simulink model "Simulation"  (Simulink 7.4)
settings: Solver=ode45  StartTime=0.0  StopTime=30.0  MaxStep=0.2  RelTol=1e-3
PostLoadFcn:
  | load StoryboardBus.mat
libraries: RailCab x2
settings Model: Creator=dread  LastModifiedBy=dread

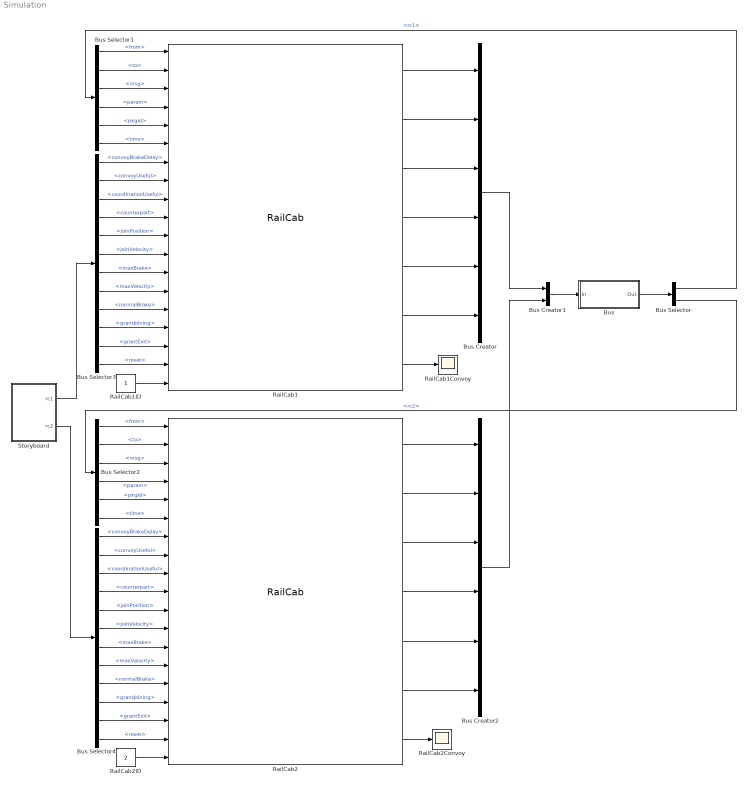
== system Simulation ==
  Bus : Subsystem
  Bus Creator : BusCreator  Inputs=6  UseBusObject=on
      settings: BusObject=PacketBus
  Bus Creator1 : BusCreator  Inputs=2  UseBusObject=on
      settings: BusObject=RailCabBus
  Bus Creator2 : BusCreator  Inputs=6  UseBusObject=on
      settings: BusObject=PacketBus
  Bus Selector : BusSelector  OutputSignals=rc1,rc2
  Bus Selector1 : BusSelector  OutputSignals=from,to,msg,param,pkgid,time
  Bus Selector2 : BusSelector  OutputSignals=from,to,msg,param,pkgid,time
  Bus Selector3 : BusSelector  OutputSignals=convoyBrakeDelay,convoyUseful,coordinationUseful,counterpart,joinPosition,joinVelocity,maxBrake,maxVelocity,normalBrake,grantJoining,grantExit,reset
  Bus Selector4 : BusSelector  OutputSignals=convoyBrakeDelay,convoyUseful,coordinationUseful,counterpart,joinPosition,joinVelocity,maxBrake,maxVelocity,normalBrake,grantJoining,grantExit,reset
  RailCab1 : RailCab/RailCab  SystemSampleTime=-1
  RailCab1Convoy : Scope
      settings: TimeRange=30
  RailCab1ID : Constant  OutDataTypeMode=uint8  OutDataType=fixdt(1, 16)  OutScaling=2^0  OutDataTypeStr=uint8
  RailCab2 : RailCab/RailCab  SystemSampleTime=-1
  RailCab2Convoy : Scope
  RailCab2ID : Constant  Value=2  OutDataTypeMode=uint8  OutDataType=fixdt(1, 16)  OutScaling=2^0  OutDataTypeStr=uint8
  Storyboard : Subsystem
  wires:
  Bus/1(Out) -> Bus Selector/1
  Bus Selector/1 -> Bus Selector1/1  "<rc1>"
  Bus Creator/1 -> Bus Creator1/1
  Bus Creator1/1 -> Bus/1(In)
  Bus Creator2/1 -> Bus Creator1/2
  Bus Selector/2 -> Bus Selector2/1  "<rc2>"
  Storyboard/1(rc1) -> Bus Selector3/1
  Storyboard/2(rc2) -> Bus Selector4/1
  Bus Selector3/1 -> RailCab1/7  "<convoyBrakeDelay>"
  Bus Selector3/2 -> RailCab1/8  "<convoyUseful>"
  Bus Selector3/3 -> RailCab1/9  "<coordinationUseful>"
  Bus Selector3/4 -> RailCab1/10  "<counterpart>"
  Bus Selector3/5 -> RailCab1/11  "<joinPosition>"
  Bus Selector3/6 -> RailCab1/12  "<joinVelocity>"
  Bus Selector3/7 -> RailCab1/13  "<maxBrake>"
  Bus Selector3/8 -> RailCab1/14  "<maxVelocity>"
  Bus Selector3/9 -> RailCab1/15  "<normalBrake>"
  Bus Selector3/10 -> RailCab1/16  "<grantJoining>"
  Bus Selector3/11 -> RailCab1/17  "<grantExit>"
  Bus Selector3/12 -> RailCab1/18  "<reset>"
  Bus Selector1/1 -> RailCab1/1  "<from>"
  Bus Selector1/2 -> RailCab1/2  "<to>"
  Bus Selector1/3 -> RailCab1/3  "<msg>"
  Bus Selector1/4 -> RailCab1/4  "<param>"
  Bus Selector1/5 -> RailCab1/5  "<pkgid>"
  Bus Selector1/6 -> RailCab1/6  "<time>"
  RailCab1/1 -> Bus Creator/1
  RailCab1/2 -> Bus Creator/2
  RailCab1/3 -> Bus Creator/3
  RailCab1/4 -> Bus Creator/4
  RailCab1/5 -> Bus Creator/5
  RailCab1/6 -> Bus Creator/6
  RailCab1ID/1 -> RailCab1/19
  Bus Selector2/1 -> RailCab2/1  "<from>"
  Bus Selector2/2 -> RailCab2/2  "<to>"
  Bus Selector2/3 -> RailCab2/3  "<msg>"
  Bus Selector2/4 -> RailCab2/4  "<param>"
  Bus Selector2/5 -> RailCab2/5  "<pkgid>"
  Bus Selector2/6 -> RailCab2/6  "<time>"
  Bus Selector4/1 -> RailCab2/7  "<convoyBrakeDelay>"
  Bus Selector4/2 -> RailCab2/8  "<convoyUseful>"
  Bus Selector4/3 -> RailCab2/9  "<coordinationUseful>"
  Bus Selector4/4 -> RailCab2/10  "<counterpart>"
  Bus Selector4/5 -> RailCab2/11  "<joinPosition>"
  Bus Selector4/6 -> RailCab2/12  "<joinVelocity>"
  Bus Selector4/7 -> RailCab2/13  "<maxBrake>"
  Bus Selector4/8 -> RailCab2/14  "<maxVelocity>"
  Bus Selector4/9 -> RailCab2/15  "<normalBrake>"
  Bus Selector4/10 -> RailCab2/16  "<grantJoining>"
  Bus Selector4/11 -> RailCab2/17  "<grantExit>"
  Bus Selector4/12 -> RailCab2/18  "<reset>"
  RailCab2ID/1 -> RailCab2/19
  RailCab2/1 -> Bus Creator2/1
  RailCab2/2 -> Bus Creator2/2
  RailCab2/3 -> Bus Creator2/3
  RailCab2/4 -> Bus Creator2/4
  RailCab2/5 -> Bus Creator2/5
  RailCab2/6 -> Bus Creator2/6
  RailCab1/7 -> RailCab1Convoy/1
  RailCab2/7 -> RailCab2Convoy/1

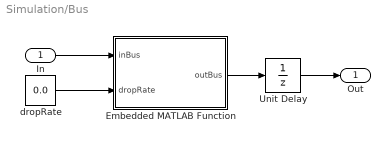
== system Simulation/Bus ==
  In : Inport  OutDataType=CommunicationBus
  Embedded MATLAB Function : Stateflow chart
  Unit Delay : UnitDelay  SampleTime=-1
  dropRate : Constant  Value=0.0  OutDataTypeMode=double  OutDataType=fixdt(1, 16)  OutScaling=2^0  OutDataTypeStr=double
  Out : Outport  OutDataType=CommunicationBus
  wires:
  Unit Delay/1 -> Out/1
  Embedded MATLAB Function/1(outBus) -> Unit Delay/1
  In/1 -> Embedded MATLAB Function/1(inBus)
  dropRate/1 -> Embedded MATLAB Function/2(dropRate)

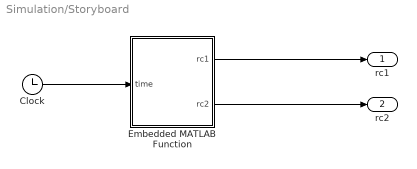
== system Simulation/Storyboard ==
  Clock : Clock
      settings: Decimation=10
  Embedded MATLAB Function : Stateflow chart
  rc1 : Outport  OutDataType=fixdt(1, 16)  OutScaling=2^0
  rc2 : Outport  Port=2  OutDataType=fixdt(1, 16)  OutScaling=2^0
  wires:
  Embedded MATLAB Function/1(rc1) -> rc1/1
  Embedded MATLAB Function/2(rc2) -> rc2/1
  Clock/1 -> Embedded MATLAB Function/1(time)

== matlab function Bus/Embedded MATLAB Function ==
  data: inBus input Bus: RailCabBus; outBus output Bus: RailCabBus; dropRate input double [0..1]
function outBus = BusImpl(inBus, dropRate)
%#eml
eml.extrinsic('fieldnames','disp','setfield','fprintf');

queueSize = 10; %length of queue
numShuttles = 0; %Define data type
numShuttles = numel(fieldnames(inBus)); %Shuttles connected to the bus
assert(numShuttles <= 20) %Defines an upper bound for number of shuttles. 
%Important for static memory allocation. 

%We need persistent queues
persistent queue

%Initialize the queues
if isempty(queue)
    queue = repmat(emptyPacket(), numShuttles, queueSize);
end

%Clean outbus
outBus = inBus;
for i = 1:numShuttles
    outBus = setfield(outBus, createRailCabName(i), emptyPacket());
end

%Retrieve packets
for i = 1:numShuttles
    packet = getPacketFromRC(inBus, i);
    if isValid(packet, numShuttles) 
        if ~dropPacket(dropRate)
            target = packet.to;
            queue(target,:) = enqueue(queue(target,:), packet);
        end
    end
end

%Send packet from queue
for i = 1:numShuttles
    if ~isEmpty(queue(i,:))
        
        %Debug: Print messages except ACK        
%         packet = front(queue(i,:));
%         if packet.msg ~= 255 %No ACK
%             fprintf('%3u: %u->%u :%3u (%.1f) @%.2f\n', packet.pkgid, packet.from, packet.to, packet.msg, packet.param, packet.time);
%         end
        
        outBus = sendPacket(outBus, front(queue(i,:)));
        queue(i,:) = dequeue(queue(i,:));                
    end    
end

%%%%%%%%%%%%%%%%%%%%%%%%%%%%%%%%%%%%%%%%%%%%%%%%%%%%%%%%%%%%%%%%%%%%%%%%%%%
%% BUS
%%%%%%%%%%%%%%%%%%%%%%%%%%%%%%%%%%%%%%%%%%%%%%%%%%%%%%%%%%%%%%%%%%%%%%%%%%%

function name = createRailCabName(index) %#eml
%Create name for the railcab used on the bus
eml.extrinsic('sprintf');
name = sprintf('rc%d', index);

function packet = getPacketFromRC(inBus, index) %#eml
%Retrieve a packet from a railcab
eml.extrinsic('getfield');
packet = emptyPacket();
packet = getfield(inBus,createRailCabName(index));

function outBus = sendPacket(outBusIn, packet) %#eml
%Send a packet to a railcab
eml.extrinsic('setfield','getfield');
outBusIn = setfield(outBusIn,createRailCabName(packet.to),packet);
outBus = outBusIn;

function drop = dropPacket(dropRate) %#eml
%Compute whether to drop the packet or not according to the given rate
eml.extrinsic('exprnd');
rand = 0;
rand = exprnd(1);
drop = rand  < -log(1-dropRate);


%%%%%%%%%%%%%%%%%%%%%%%%%%%%%%%%%%%%%%%%%%%%%%%%%%%%%%%%%%%%%%%%%%%%%%%%%%%
%% PACKET
%%%%%%%%%%%%%%%%%%%%%%%%%%%%%%%%%%%%%%%%%%%%%%%%%%%%%%%%%%%%%%%%%%%%%%%%%%%
function packet = emptyPacket() %#eml
%Creates an empty packet
packet = struct('from', uint8(0),'to', uint8(0),'msg', uint16(0),'param', double(0.0),'pkgid', uint32(0), 'time', double(0));

function valid = isValid(packet, numShuttles) %#eml
%Checks wether the given packet is valid and transported by the bus
eml.extrinsic('getfield');
valid = false;
if packet.to > 0 && packet.to <= numShuttles 
    if packet.from > 0 && packet.from <= numShuttles
        valid = true;
    end
end

%%%%%%%%%%%%%%%%%%%%%%%%%%%%%%%%%%%%%%%%%%%%%%%%%%%%%%%%%%%%%%%%%%%%%%%%%%%
%% QUEUE
%%%%%%%%%%%%%%%%%%%%%%%%%%%%%%%%%%%%%%%%%%%%%%%%%%%%%%%%%%%%%%%%%%%%%%%%%%%

function queue = enqueue(queue, packet) %#eml
%Insert the packet at the end of the queue
eml.extrinsic('warning');
for i=1:length(queue)
    if queue(i).to == 0
        queue(i) = packet;
        return;
    end
end
%No empty entry found
warning('RailCab:Bus','buffer overflow for queue %d', queue(1).to);

function queue = dequeue(queue) %#eml
%Removes the first packet of the queue
for i = 1:length(queue)-1
    queue(i) = queue(i+1);
    if queue(i).to == 0
        %end reached
        return;
    end
end
queue(length(queue)) = emptyPacket();

function packet = front(queue) %#eml
%Returns the first element from the queue
packet = queue(1);

function empty = isEmpty(queue) %#eml
%Checks whether the queue is empty or not
packet = queue(1);
if packet.to == 0
    empty = true;
else
    empty = false;
end

== matlab function Storyboard/Embedded MATLAB Function ==
  data: rc1 output Bus: StoryboardBus; rc2 output Bus: StoryboardBus; time input double
function [rc1,rc2] = storyboard(time)
%#eml
%Experimental storyboard

rc1.convoyBrakeDelay    = [0; 0; 0; 0; 7];
rc1.convoyUseful        = false;
rc1.coordinationUseful  = false;
rc1.counterpart         = 0;
rc1.joinPosition        = 0;
rc1.joinVelocity        = 100;
rc1.maxBrake            = 20;
rc1.maxVelocity         = 200;
rc1.normalBrake         = 10;
rc1.grantJoining        = false;
rc1.grantExit           = false;
rc1.reset               = false;


rc2.convoyBrakeDelay    = [0; 0; 0; 0; 7];
rc2.convoyUseful        = false;
rc2.coordinationUseful  = false;
rc2.counterpart         = 0;
rc2.joinPosition        = 0;
rc2.joinVelocity        = 100;
rc2.maxBrake            = 20;
rc2.maxVelocity         = 200;
rc2.normalBrake         = 10;
rc2.grantJoining        = false;
rc2.grantExit           = false;
rc2.reset               = false;

%Convoy formation
if 0 <= time && time < 10
    rc1.coordinationUseful  = true;
    rc1.grantJoining        = true;
    
    rc2.convoyUseful        = true;
    rc2.counterpart         = 1;
    
%Change coordinator
elseif 10 <= time && time < 20    
    rc1.coordinationUseful  = false;
    rc1.convoyUseful        = true;
    rc1.counterpart         = 2;
    
    rc2.coordinationUseful  = true;
    rc2.convoyUseful        = true;
    
%Dismiss convoy    
elseif 20 <= time && time < 30      
    rc2.coordinationUseful  = true;
    rc2.grantExit           = true;    
        
end
